simulink model "read_MPU6050_using_arduino_due"  (R2024b)
settings: Solver=FixedStepAuto  StartTime=0.0  StopTime=Inf  RelTol=1e-3  EnableMultiTasking=on
undefined symbols (not defined in the file): Discrete, Time, Ts
libraries: dspstat3 x3, simulink_extras x2, simulink x1, ctrlSharedLib x1, arduinosensorlib x1
settings Model: ExtModeTrigDuration=2  Creator=leoni  LastModifiedBy=leoni
settings SolverCC: AutoInsertRateTranBlk=on
settings OptimizationCC: EnhancedBackFolding=on  PassReuseOutputArgsAs=Individual arguments  ZeroExternalMemoryAtStartup=off  ZeroInternalMemoryAtStartup=off  MaxStackSize=64  OptimizeBlockOrder=speed  DifferentSizesBufferReuse=on  OptimizationCustomize=off  EfficientTunableParamExpr=on
settings DebuggingCC: ParameterTunabilityLossMsg=error
settings HardwareCC: ProdBitPerPointer=32  ProdBitPerSizeT=32  ProdBitPerPtrDiffT=32  ProdLargestAtomicInteger=Long  ProdLargestAtomicFloat=Double  ProdWordSize=32  ProdHWDeviceType=ARM Compatible->ARM Cortex
settings SFSimCC: MATLABDynamicMemAlloc=off
settings RTWCC: Description=Embedded Coder  SystemTargetFile=ert.tlc  HardwareBoard=Arduino Due  TemplateMakefile=ert_default_tmf  Toolchain=Arduino ARM  BuildConfiguration=Faster Runs
settings CodeAppCC: ForceParamTrailComments=on  IgnoreCustomStorageClasses=off  OperatorAnnotations=on  SimulinkDataObjDesc=on  SFDataObjDesc=on  InsertBlockDesc=on
settings ERTTargetCC: SupportContinuousTime=on  SupportVariableSizeSignals=on  ExtModeTransport=3  ExtModeStaticAlloc=on  ExtModeAutomaticAllocSize=off  ExtModeStaticAllocSize=24576  ExtModeMexFile=ext_xcp  ExtModeIntrfLevel=Level2 - Open  InlinedParameterPlacement=Hierarchical

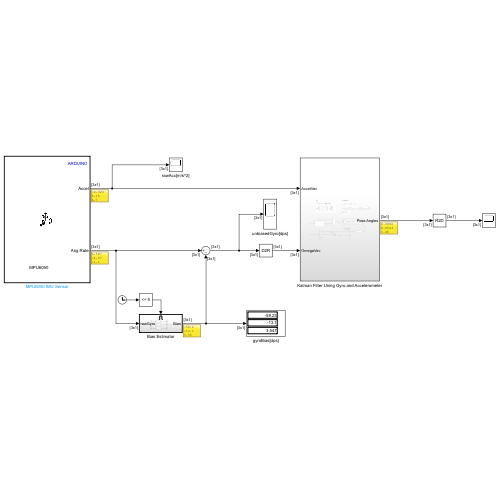
[thumbnail: Simulink's stored preview of the top-level diagram]
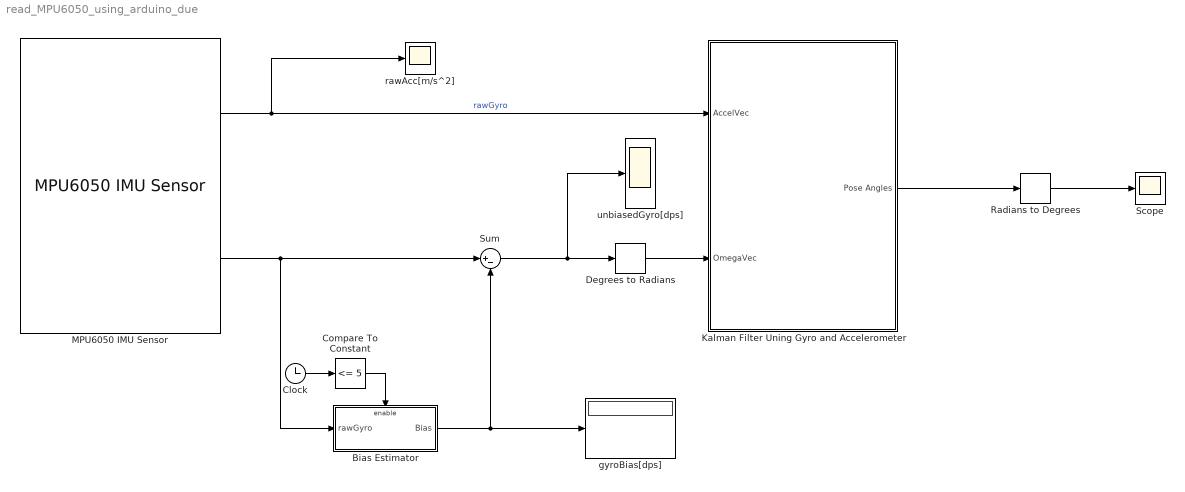
== system read_MPU6050_using_arduino_due ==
  Bias Estimator : Subsystem  TreatAsAtomicUnit=on
  Clock : Clock
  Compare To Constant : simulink/Logic and Bit Operations/Compare To Constant  relop=<=  const=5  OutDataTypeStr=boolean
  Degrees to Radians : simulink_extras/Transformations/Degrees to Radians
  Kalman Filter Uning Gyro and Accelerometer : Subsystem
  MPU6050 IMU Sensor : arduinosensorlib/MPU6050 IMU Sensor  I2CModule=0  SlaveAddress=0x68  Accel=on  AngularRate=on  Temperature=off  Status=off  Timestamp=off  EulerAngles=off  Quat=off  AccelRange=2G  GyroRange=250 dps  DmpOdr=200 Hz  Dlpf=Accelerometer: 10Hz, Gyroscope: 10Hz  spf=1  SampleTime=1/100  QueueSizeFactor=1
      settings: SourceProductName=Sensors
  Radians to Degrees : simulink_extras/Transformations/Radians to Degrees
  Scope : Scope
  Sum : Sum  Inputs=|+-
  gyroBias[dps] : Display
  rawAcc[m/s^2] : Scope
  unbiasedGyro[dps] : Scope
  wires:
  MPU6050 IMU Sensor/1 -> rawAcc[m/s^2]/1, Kalman Filter Uning Gyro and Accelerometer/1(AccelVec)  "rawGyro"
  Kalman Filter Uning Gyro and Accelerometer/1(Pose Angles) -> Radians to Degrees/1
  Radians to Degrees/1 -> Scope/1
  MPU6050 IMU Sensor/2 -> Sum/1, Bias Estimator/1(rawGyro)
  Clock/1 -> Compare To Constant/1
  Compare To Constant/1 -> Bias Estimator/Enable
  Sum/1 -> unbiasedGyro[dps]/1, Degrees to Radians/1
  Bias Estimator/1(Bias) -> gyroBias[dps]/1, Sum/2
  Degrees to Radians/1 -> Kalman Filter Uning Gyro and Accelerometer/2(OmegaVec)

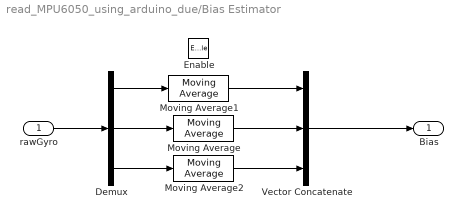
== system read_MPU6050_using_arduino_due/Bias Estimator ==
  rawGyro : Inport
  Enable : EnablePort  StatesWhenEnabling=reset
  Demux : Demux  Outputs=3
  Moving Average : dspstat3/Moving Average  Method=Exponential weighting  ForgettingFactorPort=off  SpecifyWindowLength=on  WindowLength=4  OverlapLength=3  AllowArbitraryInputLength=off  ForgettingFactor=0.9  SimulateUsing=Interpreted execution
  Moving Average1 : dspstat3/Moving Average  Method=Exponential weighting  ForgettingFactorPort=off  SpecifyWindowLength=on  WindowLength=4  OverlapLength=3  AllowArbitraryInputLength=off  ForgettingFactor=0.9  SimulateUsing=Interpreted execution
  Moving Average2 : dspstat3/Moving Average  Method=Exponential weighting  ForgettingFactorPort=off  SpecifyWindowLength=on  WindowLength=4  OverlapLength=3  AllowArbitraryInputLength=off  ForgettingFactor=0.9  SimulateUsing=Interpreted execution
  Vector Concatenate : Concatenate  NumInputs=3  Mode=Multidimensional array
  Bias : Outport
  wires:
  rawGyro/1 -> Demux/1
  Moving Average/1 -> Vector Concatenate/2
  Demux/1 -> Moving Average1/1
  Demux/2 -> Moving Average/1
  Demux/3 -> Moving Average2/1
  Moving Average2/1 -> Vector Concatenate/3
  Moving Average1/1 -> Vector Concatenate/1
  Vector Concatenate/1 -> Bias/1

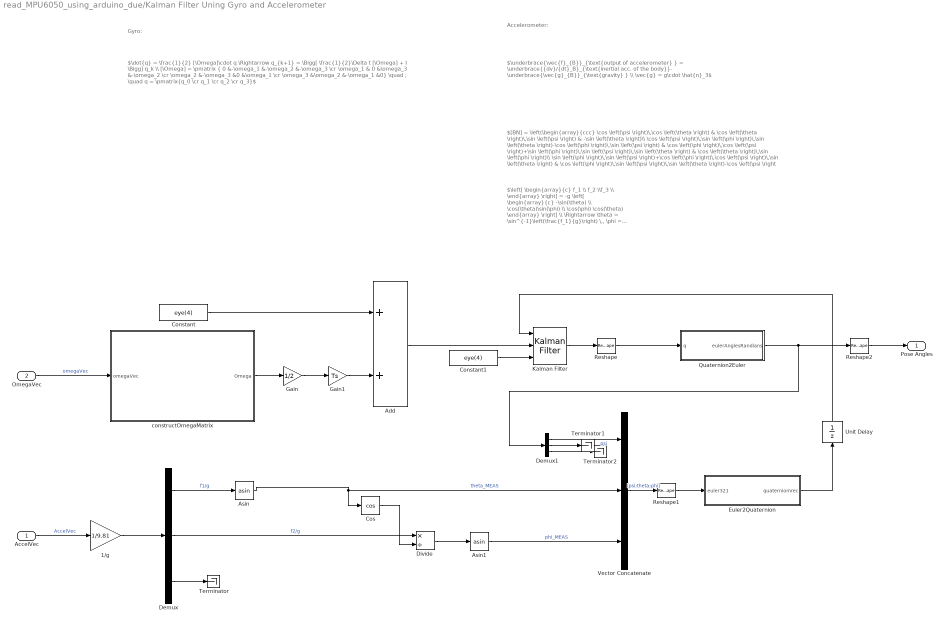
== system read_MPU6050_using_arduino_due/Kalman Filter Uning Gyro and Accelerometer ==
  note: $\left[ \begin{array}{c} f_1 \\ f_2 \\f_3 \\ \end{array} \right] = -g \left[ \begin{array}{c} -\sin(\theta) \\ \cos(\theta)\sin(\phi) \\ \cos(\phi) \cos(\theta) \end{array} \right] \\ \Rightarrow \theta = \sin^{-1}\left(\frac{f_1}{g}\right) \,, \phi = \sin^{-1} \left(\frac{-f_2}{g \cos\theta}\right)$
  note: $[BN] = \left(\begin{array}{ccc} \cos \left(\psi \right)\,\cos \left(\theta \right) & \cos \left(\theta \right)\,\sin \left(\psi \right) & -\sin \left(\theta \right)\\ \cos \left(\psi \right)\,\sin \left(\phi \right)\,\sin \left(\theta \right)-\cos \left(\phi \right)\,\sin \left(\psi \right) & \cos \left(\phi \right)\,\cos \left(\psi \right)+\sin \left(\phi \right)\,\sin \left(\psi \right)\,\sin \left(\theta \right) & \cos \left(\theta \right)\,\sin \left(\phi \right)\\ \sin \left(\phi \right)\,\sin \left(\psi \right)+\cos \left(\phi \right)\,\cos \left(\psi \right)\,\sin \left(\theta \right) & \cos \left(\phi \right)\,\sin \left(\psi \right)\,\sin \left(\theta \right)-\cos \left(\psi \right)\,\sin \left(\phi \right) & \cos \left(\phi \right)\,\cos \left(\theta \right) \end{array}\right)$
  note: $\underbrace{\vec{f}_{B}}_{\text{output of accelerometer} } = \underbrace{{dv}/{dt}_B}_{\text{inertial acc. of the body}}- \underbrace{\vec{g}_{B}}_{\text{gravity} } \\ \vec{g} = g\cdot \hat{n}_3$
  note: Gyro:
  note: $\dot{q} = \frac{1}{2} [\Omega]\cdot q \Rightarrow q_{k+1} = \Bigg[ \frac{1}{2}\Delta t [\Omega] + I \Bigg] q_k \\ [\Omega] = \pmatrix { 0 &-\omega_1 &-\omega_2 &-\omega_3 \cr \omega_1 & 0 &\omega_3 &-\omega_2 \cr \omega_2 &-\omega_3 &0 &\omega_1 \cr \omega_3 &\omega_2 &-\omega_1 &0} \quad ; \quad q = \pmatrix{q_0 \cr q_1 \cr q_2 \cr q_3}$
  note: Accelerometer:
  AccelVec : Inport  SampleTime=Ts
  OmegaVec : Inport  Port=2  SampleTime=Ts
  1/g : Gain  Gain=1/9.81
  Add : Sum
  Asin : Trigonometry  Operator=asin
  Asin1 : Trigonometry  Operator=asin
  Constant : Constant  Value=eye(4)  SampleTime=Ts
  Constant1 : Constant  Value=eye(4)  SampleTime=Ts
  Cos : Trigonometry  Operator=cos
  Demux : Demux  Outputs=3
  Demux1 : Demux  Outputs=3
  Divide : Product  Inputs=*/
  Euler2Quaternion : MATLAB Function  TreatAsAtomicUnit=on
  Gain : Gain  Gain=1/2
  Gain1 : Gain  Gain=Ts
  Kalman Filter : ctrlSharedLib/Kalman Filter  TimeDomain=Discrete-Time  UseCurrentEstimator=on  ModelSource=Input port  ModelSourceVariable=ss(0.95,1,1,0,1)  A=0.95  B=1  C=1  D=0  NumberOfStates=4  NumberOfInputs=1  NumberOfOutputs=4  InitialEstimateSource=Dialog  X0=[1;0;0;0]  P0=eye(4)  UseK=off  UseGH=off  NumberOfProcessNoiseInputs=1  G=1  TimeInvariantG=on  H=0  TimeInvariantH=on  Q=0.001*eye(4)  TimeInvariantQ=on  R=10*eye(4)  TimeInvariantR=on  N=0  TimeInvariantN=on  AddInputPort=off  AddEnablePort=off  OutputEstimatedY=off  OutputP=off  Ts=Ts
  Quaternion2Euler : MATLAB Function  TreatAsAtomicUnit=on
  Reshape : Reshape  OutputDimensionality=Column vector (2-D)
  Reshape1 : Reshape  OutputDimensionality=Row vector (2-D)
  Reshape2 : Reshape  OutputDimensionality=Column vector (2-D)
  Terminator : Terminator
  Terminator1 : Terminator
  Terminator2 : Terminator
  Unit Delay : UnitDelay  SampleTime=-1  HasFrameUpgradeWarning=on
  Vector Concatenate : Concatenate  NumInputs=3  Mode=Multidimensional array
  constructOmegaMatrix : MATLAB Function  TreatAsAtomicUnit=on
  Pose Angles : Outport  SampleTime=Ts
  wires:
  Reshape/1 -> Quaternion2Euler/1(q)
  Constant1/1 -> Kalman Filter/3
  Add/1 -> Kalman Filter/2
  Constant/1 -> Add/1
  Gain/1 -> Gain1/1
  Gain1/1 -> Add/2
  Kalman Filter/1 -> Reshape/1
  constructOmegaMatrix/1(Omega) -> Gain/1
  OmegaVec/1 -> constructOmegaMatrix/1(omegaVec)  "omegaVec"
  AccelVec/1 -> 1/g/1  "AccelVec"
  Demux/1 -> Asin/1  "f1/g"
  Demux/2 -> Divide/1  "f2/g"
  1/g/1 -> Demux/1
  Demux/3 -> Terminator/1
  Asin/1 -> Cos/1, Vector Concatenate/2  "theta_MEAS"
  Cos/1 -> Divide/2
  Divide/1 -> Asin1/1
  Asin1/1 -> Vector Concatenate/3  "phi_MEAS"
  Vector Concatenate/1 -> Reshape1/1  "[psi;theta;phi]"
  Demux1/2 -> Terminator1/1
  Demux1/3 -> Terminator2/1
  Demux1/1 -> Vector Concatenate/1  "psi"
  Euler2Quaternion/1(quaternionVec) -> Unit Delay/1
  Unit Delay/1 -> Kalman Filter/1
  Quaternion2Euler/1(eulerAnglesRandians) -> Demux1/1, Reshape2/1
  Reshape1/1 -> Euler2Quaternion/1(euler321)
  Reshape2/1 -> Pose Angles/1

== matlab function read_MPU6050_using_arduino_due/Kalman Filter Uning Gyro and Accelerometer/constructOmegaMatrix ==
  data: omegaVec input; Omega output
function  Omega = fcn(omegaVec)

w1 = omegaVec(1);
w2 = omegaVec(2);
w3 = omegaVec(3);


Omega = [0 -w1 -w2 -w3;...
         w1 0   w3 -w2;...
         w2 -w3 0 w1;...
         w3 w2 -w1 0];

== matlab function read_MPU6050_using_arduino_due/Kalman Filter Uning Gyro and Accelerometer/Euler2Quaternion ==
  data: euler321 input; quaternionVec output
function quaternionVec = fcn(euler321)


quaternionVec =  compact(quaternion(euler321,"euler","ZYX","frame"));

end

== matlab function read_MPU6050_using_arduino_due/Kalman Filter Uning Gyro and Accelerometer/Quaternion2Euler ==
  data: q input; eulerAnglesRandians output
function eulerAnglesRandians = fcn(q)

quat = quaternion([q(1) q(2) q(3) q(4)]);

eulerAnglesRandians = euler(quat,"ZYX","frame");

end
